simulink model "EPT"  (R2019b)
settings: Solver=FixedStepDiscrete  StartTime=0.0  StopTime=5  FixedStep=0.005  RelTol=1e-3  EnableMultiTasking=on
PreLoadFcn:
  | try, model_open; catch, disp('Error occurred while executing model pre-load callback: model_open.m'); disp('Please assure that the MATLAB working directory is set to the model directory before opening.'); end
InitFcn:
  | try, model_open; catch, end
undefined symbols (not defined in the file or in its folder): Bridge, GCM, H, ln, raptor_get_param_eval, raptor_get_safe_string, raptor_xcp_function
libraries: Raptor_lib x2810, simulink x374, hdlsllib x19
(part 26 of 45)

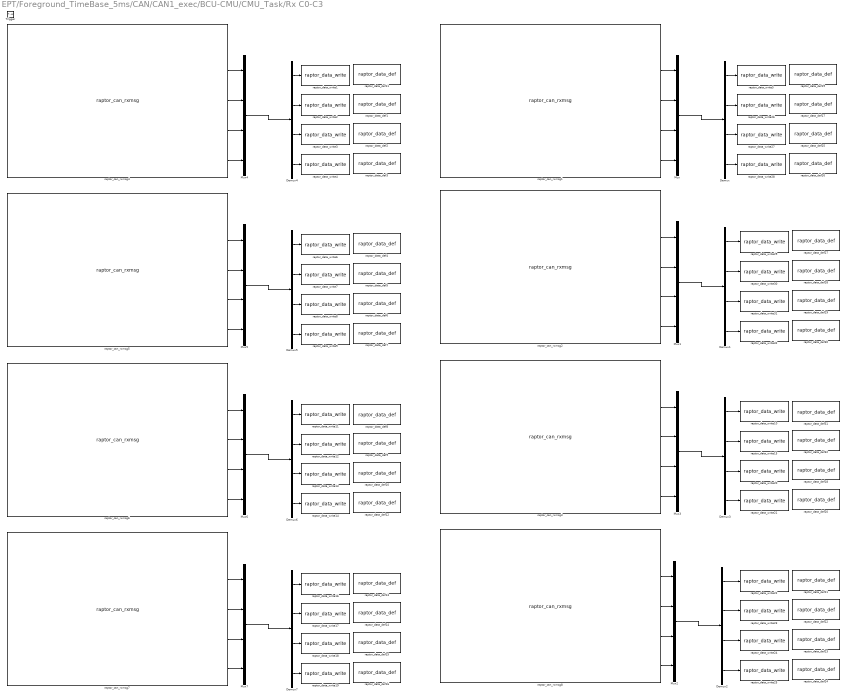
== system EPT/Foreground_TimeBase_5ms/CAN/CAN1_exec/BCU-CMU/CMU_Task/Rx C0-C3 ==
  Trigger : TriggerPort  VariantControl=Variant  PortDimensions=1
  Demux{,1..7} (8 alike) : Demux
  Mux{,1..7} (8 alike) : Mux
  raptor_can_rxmsg1 : Raptor_lib/CAN/raptor_can_rxmsg  canDefinition=struct('dbcFile', 'CMU2.dbc','message', 'Cell_Volt1','comment', '','signals', {{'Vcell1','Vcell2','Vcell3','Vcell4'}},'enabled', [ 1 1 1 1;],'canBus', '''CAN1''','messageID', [ 33603746;],'idMask', [ 536870911;],'payloadMask', [],'payloadValue', [],'period', [ 0;],'mailbox', '''''','queueSize', [ 1;],'label', [ 0;],'ver', [ 2;],'showID', [ 0;],'showRaw', [ 0;],'fill', [ 0;],'editID', [ 0;],'signalOrder', [ 2;])  canBus='CAN1'  mailbox=''  payloadMask=[]  payloadValue=[]  idMask=hex2dec('1FFFFFFF')  queueSize=1  showID=0  label=0  fill=0  id=33603746  showRaw=0  showAge=1  signalOrder=2  signalInfo={{struct('Name', 'Vcell1','Startbit', [ 0;],'SignalSize', [ 16;],'ByteOrder', 'BigEndian','ValueType', 'UNSIGNED','Class', 'uint16','Signed', [ 0;],'Factor', [ 0.001;],'Offset', [ 0;],'Min', [ 0;],'Max', [ 0;],'Units', '','Comment', '','StartBit', [ 8;]),struct('Name', 'Vcell2','Startbit', [ 0;],'SignalSize', [ 16;],'ByteOrder', 'BigEndian','ValueType', 'UNSIGNED','Class', 'uint16','Signed', [ 0;],'Factor', [ 0.001;],'Offset', [ 0;],'Min', [ 0;],'Max', [ 0;],'Units', '','Comment', '','StartBit', [ 24;]),struct('Name', 'Vcell3','Startbit', [ 0;],'SignalSize', [ 16;],'ByteOrder', 'BigEndian','ValueType', 'UNSIGNED','Class', 'uint16','Signed', [ 0;],'Factor', [ 0.001;],'Offset', [ 0;],'Min', [ 0;],'Max', [ 0;],'Units', '','Comment', '','StartBit', [ 40;]),struct('Name', 'Vcell4','Startbit', [ 0;],'SignalSize', [ 16;],'ByteOrder', 'BigEndian','ValueType', 'UNSIGNED','Class', 'uint16','Signed', [ 0;],'Factor', [ 0.001;],'Offset', [ 0;],'Min', [ 0;],'Max', [ 0;],'Units', '','Comment', '','StartBit', [ 56;])}}
      settings: SourceProductName=Raptor
  raptor_can_rxmsg2 : Raptor_lib/CAN/raptor_can_rxmsg  canDefinition=struct('dbcFile', 'CMU2.dbc','message', 'Cell_Volt2','comment', '','signals', {{'Vcell5','Vcell6','Vcell7','Vcell8'}},'enabled', [ 1 1 1 1;],'canBus', '''CAN1''','messageID', [ 33604002;],'idMask', [ 536870911;],'payloadMask', [],'payloadValue', [],'period', [ 0;],'mailbox', '''''','queueSize', [ 1;],'label', [ 0;],'ver', [ 2;],'showID', [ 0;],'showRaw', [ 0;],'fill', [ 0;],'editID', [ 0;],'signalOrder', [ 2;])  canBus='CAN1'  mailbox=''  payloadMask=[]  payloadValue=[]  idMask=hex2dec('1FFFFFFF')  queueSize=1  showID=0  label=0  fill=0  id=33604002  showRaw=0  showAge=1  signalOrder=2  signalInfo={{struct('Name', 'Vcell5','Startbit', [ 0;],'SignalSize', [ 16;],'ByteOrder', 'BigEndian','ValueType', 'UNSIGNED','Class', 'uint16','Signed', [ 0;],'Factor', [ 0.001;],'Offset', [ 0;],'Min', [ 0;],'Max', [ 0;],'Units', '','Comment', '','StartBit', [ 8;]),struct('Name', 'Vcell6','Startbit', [ 0;],'SignalSize', [ 16;],'ByteOrder', 'BigEndian','ValueType', 'UNSIGNED','Class', 'uint16','Signed', [ 0;],'Factor', [ 0.001;],'Offset', [ 0;],'Min', [ 0;],'Max', [ 0;],'Units', '','Comment', '','StartBit', [ 24;]),struct('Name', 'Vcell7','Startbit', [ 0;],'SignalSize', [ 16;],'ByteOrder', 'BigEndian','ValueType', 'UNSIGNED','Class', 'uint16','Signed', [ 0;],'Factor', [ 0.001;],'Offset', [ 0;],'Min', [ 0;],'Max', [ 0;],'Units', '','Comment', '','StartBit', [ 40;]),struct('Name', 'Vcell8','Startbit', [ 0;],'SignalSize', [ 16;],'ByteOrder', 'BigEndian','ValueType', 'UNSIGNED','Class', 'uint16','Signed', [ 0;],'Factor', [ 0.001;],'Offset', [ 0;],'Min', [ 0;],'Max', [ 0;],'Units', '','Comment', '','StartBit', [ 56;])}}
      settings: SourceProductName=Raptor
  raptor_can_rxmsg3 : Raptor_lib/CAN/raptor_can_rxmsg  canDefinition=struct('dbcFile', 'CMU2.dbc','message', 'Cell_Volt3','comment', '','signals', {{'Vcell9','Vcell10','Vcell11','Vcell12'}},'enabled', [ 1 1 1 1;],'canBus', '''CAN1''','messageID', [ 33604258;],'idMask', [ 536870911;],'payloadMask', [],'payloadValue', [],'period', [ 0;],'mailbox', '''''','queueSize', [ 1;],'label', [ 0;],'ver', [ 2;],'showID', [ 0;],'showRaw', [ 0;],'fill', [ 0;],'editID', [ 0;],'signalOrder', [ 2;])  canBus='CAN1'  mailbox=''  payloadMask=[]  payloadValue=[]  idMask=hex2dec('1FFFFFFF')  queueSize=1  showID=0  label=0  fill=0  id=33604258  showRaw=0  showAge=1  signalOrder=2  signalInfo={{struct('Name', 'Vcell9','Startbit', [ 0;],'SignalSize', [ 16;],'ByteOrder', 'BigEndian','ValueType', 'UNSIGNED','Class', 'uint16','Signed', [ 0;],'Factor', [ 0.001;],'Offset', [ 0;],'Min', [ 0;],'Max', [ 0;],'Units', '','Comment', '','StartBit', [ 8;]),struct('Name', 'Vcell10','Startbit', [ 0;],'SignalSize', [ 16;],'ByteOrder', 'BigEndian','ValueType', 'UNSIGNED','Class', 'uint16','Signed', [ 0;],'Factor', [ 0.001;],'Offset', [ 0;],'Min', [ 0;],'Max', [ 0;],'Units', '','Comment', '','StartBit', [ 24;]),struct('Name', 'Vcell11','Startbit', [ 0;],'SignalSize', [ 16;],'ByteOrder', 'BigEndian','ValueType', 'UNSIGNED','Class', 'uint16','Signed', [ 0;],'Factor', [ 0.001;],'Offset', [ 0;],'Min', [ 0;],'Max', [ 0;],'Units', '','Comment', '','StartBit', [ 40;]),struct('Name', 'Vcell12','Startbit', [ 0;],'SignalSize', [ 16;],'ByteOrder', 'BigEndian','ValueType', 'UNSIGNED','Class', 'uint16','Signed', [ 0;],'Factor', [ 0.001;],'Offset', [ 0;],'Min', [ 0;],'Max', [ 0;],'Units', '','Comment', '','StartBit', [ 56;])}}
      settings: SourceProductName=Raptor
  raptor_can_rxmsg4 : Raptor_lib/CAN/raptor_can_rxmsg  canDefinition=struct('dbcFile', 'CMU1.dbc','message', 'Cell_Volt1','comment', '','signals', {{'Vcell1','Vcell2','Vcell3','Vcell4'}},'enabled', [ 1 1 1 1;],'canBus', '''CAN1''','messageID', [ 33603745;],'idMask', [ 536870911;],'payloadMask', [],'payloadValue', [],'period', [ 0;],'mailbox', '''''','queueSize', [ 1;],'label', [ 0;],'ver', [ 2;],'showID', [ 0;],'showRaw', [ 0;],'fill', [ 0;],'editID', [ 0;],'signalOrder', [ 2;])  canBus='CAN1'  mailbox=''  payloadMask=[]  payloadValue=[]  idMask=hex2dec('1FFFFFFF')  queueSize=1  showID=0  label=0  fill=0  id=33603745  showRaw=0  showAge=1  signalOrder=2  signalInfo={{struct('Name', 'Vcell1','Startbit', [ 0;],'SignalSize', [ 16;],'ByteOrder', 'BigEndian','ValueType', 'UNSIGNED','Class', 'uint16','Signed', [ 0;],'Factor', [ 0.001;],'Offset', [ 0;],'Min', [ 0;],'Max', [ 0;],'Units', '','Comment', '','StartBit', [ 8;]),struct('Name', 'Vcell2','Startbit', [ 0;],'SignalSize', [ 16;],'ByteOrder', 'BigEndian','ValueType', 'UNSIGNED','Class', 'uint16','Signed', [ 0;],'Factor', [ 0.001;],'Offset', [ 0;],'Min', [ 0;],'Max', [ 0;],'Units', '','Comment', '','StartBit', [ 24;]),struct('Name', 'Vcell3','Startbit', [ 0;],'SignalSize', [ 16;],'ByteOrder', 'BigEndian','ValueType', 'UNSIGNED','Class', 'uint16','Signed', [ 0;],'Factor', [ 0.001;],'Offset', [ 0;],'Min', [ 0;],'Max', [ 0;],'Units', '','Comment', '','StartBit', [ 40;]),struct('Name', 'Vcell4','Startbit', [ 0;],'SignalSize', [ 16;],'ByteOrder', 'BigEndian','ValueType', 'UNSIGNED','Class', 'uint16','Signed', [ 0;],'Factor', [ 0.001;],'Offset', [ 0;],'Min', [ 0;],'Max', [ 0;],'Units', '','Comment', '','StartBit', [ 56;])}}
      settings: SourceProductName=Raptor
  raptor_can_rxmsg5 : Raptor_lib/CAN/raptor_can_rxmsg  canDefinition=struct('dbcFile', 'CMU1.dbc','message', 'Cell_Volt2','comment', '','signals', {{'Vcell5','Vcell6','Vcell7','Vcell8'}},'enabled', [ 1 1 1 1;],'canBus', '''CAN1''','messageID', [ 33604001;],'idMask', [ 536870911;],'payloadMask', [],'payloadValue', [],'period', [ 0;],'mailbox', '''''','queueSize', [ 1;],'label', [ 0;],'ver', [ 2;],'showID', [ 0;],'showRaw', [ 0;],'fill', [ 0;],'editID', [ 0;],'signalOrder', [ 2;])  canBus='CAN1'  mailbox=''  payloadMask=[]  payloadValue=[]  idMask=hex2dec('1FFFFFFF')  queueSize=1  showID=0  label=0  fill=0  id=33604001  showRaw=0  showAge=1  signalOrder=2  signalInfo={{struct('Name', 'Vcell5','Startbit', [ 0;],'SignalSize', [ 16;],'ByteOrder', 'BigEndian','ValueType', 'UNSIGNED','Class', 'uint16','Signed', [ 0;],'Factor', [ 0.001;],'Offset', [ 0;],'Min', [ 0;],'Max', [ 0;],'Units', '','Comment', '','StartBit', [ 8;]),struct('Name', 'Vcell6','Startbit', [ 0;],'SignalSize', [ 16;],'ByteOrder', 'BigEndian','ValueType', 'UNSIGNED','Class', 'uint16','Signed', [ 0;],'Factor', [ 0.001;],'Offset', [ 0;],'Min', [ 0;],'Max', [ 0;],'Units', '','Comment', '','StartBit', [ 24;]),struct('Name', 'Vcell7','Startbit', [ 0;],'SignalSize', [ 16;],'ByteOrder', 'BigEndian','ValueType', 'UNSIGNED','Class', 'uint16','Signed', [ 0;],'Factor', [ 0.001;],'Offset', [ 0;],'Min', [ 0;],'Max', [ 0;],'Units', '','Comment', '','StartBit', [ 40;]),struct('Name', 'Vcell8','Startbit', [ 0;],'SignalSize', [ 16;],'ByteOrder', 'BigEndian','ValueType', 'UNSIGNED','Class', 'uint16','Signed', [ 0;],'Factor', [ 0.001;],'Offset', [ 0;],'Min', [ 0;],'Max', [ 0;],'Units', '','Comment', '','StartBit', [ 56;])}}
      settings: SourceProductName=Raptor
  raptor_can_rxmsg6 : Raptor_lib/CAN/raptor_can_rxmsg  canDefinition=struct('dbcFile', 'CMU1.dbc','message', 'Cell_Volt3','comment', '','signals', {{'Vcell9','Vcell10','Vcell11','Vcell12'}},'enabled', [ 1 1 1 1;],'canBus', '''CAN1''','messageID', [ 33604257;],'idMask', [ 536870911;],'payloadMask', [],'payloadValue', [],'period', [ 0;],'mailbox', '''''','queueSize', [ 1;],'label', [ 0;],'ver', [ 2;],'showID', [ 0;],'showRaw', [ 0;],'fill', [ 0;],'editID', [ 0;],'signalOrder', [ 3;])  canBus='CAN1'  mailbox=''  payloadMask=[]  payloadValue=[]  idMask=hex2dec('1FFFFFFF')  queueSize=1  showID=0  label=0  fill=0  id=33604257  showRaw=0  showAge=1  signalOrder=3  signalInfo={{struct('Name', 'Vcell9','Startbit', [ 0;],'SignalSize', [ 16;],'ByteOrder', 'BigEndian','ValueType', 'UNSIGNED','Class', 'uint16','Signed', [ 0;],'Factor', [ 0.001;],'Offset', [ 0;],'Min', [ 0;],'Max', [ 0;],'Units', '','Comment', '','StartBit', [ 8;]),struct('Name', 'Vcell10','Startbit', [ 0;],'SignalSize', [ 16;],'ByteOrder', 'BigEndian','ValueType', 'UNSIGNED','Class', 'uint16','Signed', [ 0;],'Factor', [ 0.001;],'Offset', [ 0;],'Min', [ 0;],'Max', [ 0;],'Units', '','Comment', '','StartBit', [ 24;]),struct('Name', 'Vcell11','Startbit', [ 0;],'SignalSize', [ 16;],'ByteOrder', 'BigEndian','ValueType', 'UNSIGNED','Class', 'uint16','Signed', [ 0;],'Factor', [ 0.001;],'Offset', [ 0;],'Min', [ 0;],'Max', [ 0;],'Units', '','Comment', '','StartBit', [ 40;]),struct('Name', 'Vcell12','Startbit', [ 0;],'SignalSize', [ 16;],'ByteOrder', 'BigEndian','ValueType', 'UNSIGNED','Class', 'uint16','Signed', [ 0;],'Factor', [ 0.001;],'Offset', [ 0;],'Min', [ 0;],'Max', [ 0;],'Units', '','Comment', '','StartBit', [ 56;])}}
      settings: SourceProductName=Raptor
  raptor_can_rxmsg7 : Raptor_lib/CAN/raptor_can_rxmsg  canDefinition=struct('dbcFile', 'CMU1.dbc','message', 'Cell_Volt4','comment', '','signals', {{'Vcell13','Vcell14','Vcell15','Vcell16'}},'enabled', [ 1 1 1 1;],'canBus', '''CAN1''','messageID', [ 33604513;],'idMask', [ 536870911;],'payloadMask', [],'payloadValue', [],'period', [ 0;],'mailbox', '''''','queueSize', [ 1;],'label', [ 0;],'ver', [ 2;],'showID', [ 0;],'showRaw', [ 0;],'fill', [ 0;],'editID', [ 0;],'signalOrder', [ 2;])  canBus='CAN1'  mailbox=''  payloadMask=[]  payloadValue=[]  idMask=hex2dec('1FFFFFFF')  queueSize=1  showID=0  label=0  fill=0  id=33604513  showRaw=0  showAge=1  signalOrder=2  signalInfo={{struct('Name', 'Vcell13','Startbit', [ 0;],'SignalSize', [ 16;],'ByteOrder', 'BigEndian','ValueType', 'UNSIGNED','Class', 'uint16','Signed', [ 0;],'Factor', [ 0.001;],'Offset', [ 0;],'Min', [ 0;],'Max', [ 0;],'Units', '','Comment', '','StartBit', [ 8;]),struct('Name', 'Vcell14','Startbit', [ 0;],'SignalSize', [ 16;],'ByteOrder', 'BigEndian','ValueType', 'UNSIGNED','Class', 'uint16','Signed', [ 0;],'Factor', [ 0.001;],'Offset', [ 0;],'Min', [ 0;],'Max', [ 0;],'Units', '','Comment', '','StartBit', [ 24;]),struct('Name', 'Vcell15','Startbit', [ 0;],'SignalSize', [ 16;],'ByteOrder', 'BigEndian','ValueType', 'UNSIGNED','Class', 'uint16','Signed', [ 0;],'Factor', [ 0.001;],'Offset', [ 0;],'Min', [ 0;],'Max', [ 0;],'Units', '','Comment', '','StartBit', [ 40;]),struct('Name', 'Vcell16','Startbit', [ 0;],'SignalSize', [ 16;],'ByteOrder', 'BigEndian','ValueType', 'UNSIGNED','Class', 'uint16','Signed', [ 0;],'Factor', [ 0.001;],'Offset', [ 0;],'Min', [ 0;],'Max', [ 0;],'Units', '','Comment', '','StartBit', [ 56;])}}
      settings: SourceProductName=Raptor
  raptor_can_rxmsg8 : Raptor_lib/CAN/raptor_can_rxmsg  canDefinition=struct('dbcFile', 'CMU2.dbc','message', 'Cell_Volt4','comment', '','signals', {{'Vcell13','Vcell14','Vcell15','Vcell16'}},'enabled', [ 1 1 1 1;],'canBus', '''CAN1''','messageID', [ 33604514;],'idMask', [ 536870911;],'payloadMask', [],'payloadValue', [],'period', [ 0;],'mailbox', '''''','queueSize', [ 1;],'label', [ 0;],'ver', [ 2;],'showID', [ 0;],'showRaw', [ 0;],'fill', [ 0;],'editID', [ 0;],'signalOrder', [ 2;])  canBus='CAN1'  mailbox=''  payloadMask=[]  payloadValue=[]  idMask=hex2dec('1FFFFFFF')  queueSize=1  showID=0  label=0  fill=0  id=33604514  showRaw=0  showAge=1  signalOrder=2  signalInfo={{struct('Name', 'Vcell13','Startbit', [ 0;],'SignalSize', [ 16;],'ByteOrder', 'BigEndian','ValueType', 'UNSIGNED','Class', 'uint16','Signed', [ 0;],'Factor', [ 0.001;],'Offset', [ 0;],'Min', [ 0;],'Max', [ 0;],'Units', '','Comment', '','StartBit', [ 8;]),struct('Name', 'Vcell14','Startbit', [ 0;],'SignalSize', [ 16;],'ByteOrder', 'BigEndian','ValueType', 'UNSIGNED','Class', 'uint16','Signed', [ 0;],'Factor', [ 0.001;],'Offset', [ 0;],'Min', [ 0;],'Max', [ 0;],'Units', '','Comment', '','StartBit', [ 24;]),struct('Name', 'Vcell15','Startbit', [ 0;],'SignalSize', [ 16;],'ByteOrder', 'BigEndian','ValueType', 'UNSIGNED','Class', 'uint16','Signed', [ 0;],'Factor', [ 0.001;],'Offset', [ 0;],'Min', [ 0;],'Max', [ 0;],'Units', '','Comment', '','StartBit', [ 40;]),struct('Name', 'Vcell16','Startbit', [ 0;],'SignalSize', [ 16;],'ByteOrder', 'BigEndian','ValueType', 'UNSIGNED','Class', 'uint16','Signed', [ 0;],'Factor', [ 0.001;],'Offset', [ 0;],'Min', [ 0;],'Max', [ 0;],'Units', '','Comment', '','StartBit', [ 56;])}}
      settings: SourceProductName=Raptor
  raptor_data_def1 : Raptor_lib/Data Storage/raptor_data_def  dataName='CMU1_CELL02_VOLT'  initValue=0  dataType=double  storage=Volatile (RAM)  calVisible=on  calType=Adjustment  calDispType=Number  calEnum={'False', 'True'}  calGain=1.0  calOffset=0  calMin=-inf  calMax=inf  calFormat='2.3'  calUnit=''  calHelp=''  calAccess=1  calFunction=raptor_xcp_function(gcb)  calDispHeaders=off  calColHeaders={'Col1' 'Col2' 'Col3'}  calRowHeaders={'Row1' 'Row2' 'Row3'}
      settings: SourceProductName=Raptor
  raptor_data_def10 : Raptor_lib/Data Storage/raptor_data_def  dataName='CMU1_CELL11_VOLT'  initValue=0  dataType=double  storage=Volatile (RAM)  calVisible=on  calType=Adjustment  calDispType=Number  calEnum={'False', 'True'}  calGain=1.0  calOffset=0  calMin=-inf  calMax=inf  calFormat='2.3'  calUnit=''  calHelp=''  calAccess=1  calFunction=raptor_xcp_function(gcb)  calDispHeaders=off  calColHeaders={'Col1' 'Col2' 'Col3'}  calRowHeaders={'Row1' 'Row2' 'Row3'}
      settings: SourceProductName=Raptor
  raptor_data_def11 : Raptor_lib/Data Storage/raptor_data_def  dataName='CMU1_CELL01_VOLT'  initValue=0  dataType=double  storage=Volatile (RAM)  calVisible=on  calType=Adjustment  calDispType=Number  calEnum={'False', 'True'}  calGain=1.0  calOffset=0  calMin=-inf  calMax=inf  calFormat='2.3'  calUnit=''  calHelp=''  calAccess=1  calFunction=raptor_xcp_function(gcb)  calDispHeaders=off  calColHeaders={'Col1' 'Col2' 'Col3'}  calRowHeaders={'Row1' 'Row2' 'Row3'}
      settings: SourceProductName=Raptor
  raptor_data_def12 : Raptor_lib/Data Storage/raptor_data_def  dataName='CMU1_CELL12_VOLT'  initValue=0  dataType=double  storage=Volatile (RAM)  calVisible=on  calType=Adjustment  calDispType=Number  calEnum={'False', 'True'}  calGain=1.0  calOffset=0  calMin=-inf  calMax=inf  calFormat='2.3'  calUnit=''  calHelp=''  calAccess=1  calFunction=raptor_xcp_function(gcb)  calDispHeaders=off  calColHeaders={'Col1' 'Col2' 'Col3'}  calRowHeaders={'Row1' 'Row2' 'Row3'}
      settings: SourceProductName=Raptor
  raptor_data_def13 : Raptor_lib/Data Storage/raptor_data_def  dataName='CMU1_CELL13_VOLT'  initValue=0  dataType=double  storage=Volatile (RAM)  calVisible=on  calType=Adjustment  calDispType=Number  calEnum={'False', 'True'}  calGain=1.0  calOffset=0  calMin=-inf  calMax=inf  calFormat='2.3'  calUnit=''  calHelp=''  calAccess=1  calFunction=raptor_xcp_function(gcb)  calDispHeaders=off  calColHeaders={'Col1' 'Col2' 'Col3'}  calRowHeaders={'Row1' 'Row2' 'Row3'}
      settings: SourceProductName=Raptor
  raptor_data_def14 : Raptor_lib/Data Storage/raptor_data_def  dataName='CMU1_CELL14_VOLT'  initValue=0  dataType=double  storage=Volatile (RAM)  calVisible=on  calType=Adjustment  calDispType=Number  calEnum={'False', 'True'}  calGain=1.0  calOffset=0  calMin=-inf  calMax=inf  calFormat='2.3'  calUnit=''  calHelp=''  calAccess=1  calFunction=raptor_xcp_function(gcb)  calDispHeaders=off  calColHeaders={'Col1' 'Col2' 'Col3'}  calRowHeaders={'Row1' 'Row2' 'Row3'}
      settings: SourceProductName=Raptor
  raptor_data_def15 : Raptor_lib/Data Storage/raptor_data_def  dataName='CMU1_CELL15_VOLT'  initValue=0  dataType=double  storage=Volatile (RAM)  calVisible=on  calType=Adjustment  calDispType=Number  calEnum={'False', 'True'}  calGain=1.0  calOffset=0  calMin=-inf  calMax=inf  calFormat='2.3'  calUnit=''  calHelp=''  calAccess=1  calFunction=raptor_xcp_function(gcb)  calDispHeaders=off  calColHeaders={'Col1' 'Col2' 'Col3'}  calRowHeaders={'Row1' 'Row2' 'Row3'}
      settings: SourceProductName=Raptor
  raptor_data_def16 : Raptor_lib/Data Storage/raptor_data_def  dataName='CMU1_CELL16_VOLT'  initValue=0  dataType=double  storage=Volatile (RAM)  calVisible=on  calType=Adjustment  calDispType=Number  calEnum={'False', 'True'}  calGain=1.0  calOffset=0  calMin=-inf  calMax=inf  calFormat='2.3'  calUnit=''  calHelp=''  calAccess=1  calFunction=raptor_xcp_function(gcb)  calDispHeaders=off  calColHeaders={'Col1' 'Col2' 'Col3'}  calRowHeaders={'Row1' 'Row2' 'Row3'}
      settings: SourceProductName=Raptor
  raptor_data_def17 : Raptor_lib/Data Storage/raptor_data_def  dataName='CMU2_CELL02_VOLT'  initValue=0  dataType=double  storage=Volatile (RAM)  calVisible=on  calType=Adjustment  calDispType=Number  calEnum={'False', 'True'}  calGain=1.0  calOffset=0  calMin=-inf  calMax=inf  calFormat='2.3'  calUnit=''  calHelp=''  calAccess=1  calFunction=raptor_xcp_function(gcb)  calDispHeaders=off  calColHeaders={'Col1' 'Col2' 'Col3'}  calRowHeaders={'Row1' 'Row2' 'Row3'}
      settings: SourceProductName=Raptor
  raptor_data_def18 : Raptor_lib/Data Storage/raptor_data_def  dataName='CMU2_CELL11_VOLT'  initValue=0  dataType=double  storage=Volatile (RAM)  calVisible=on  calType=Adjustment  calDispType=Number  calEnum={'False', 'True'}  calGain=1.0  calOffset=0  calMin=-inf  calMax=inf  calFormat='2.3'  calUnit=''  calHelp=''  calAccess=1  calFunction=raptor_xcp_function(gcb)  calDispHeaders=off  calColHeaders={'Col1' 'Col2' 'Col3'}  calRowHeaders={'Row1' 'Row2' 'Row3'}
      settings: SourceProductName=Raptor
  raptor_data_def19 : Raptor_lib/Data Storage/raptor_data_def  dataName='CMU2_CELL01_VOLT'  initValue=0  dataType=double  storage=Volatile (RAM)  calVisible=on  calType=Adjustment  calDispType=Number  calEnum={'False', 'True'}  calGain=1.0  calOffset=0  calMin=-inf  calMax=inf  calFormat='2.3'  calUnit=''  calHelp=''  calAccess=1  calFunction=raptor_xcp_function(gcb)  calDispHeaders=off  calColHeaders={'Col1' 'Col2' 'Col3'}  calRowHeaders={'Row1' 'Row2' 'Row3'}
      settings: SourceProductName=Raptor
  raptor_data_def2 : Raptor_lib/Data Storage/raptor_data_def  dataName='CMU1_CELL03_VOLT'  initValue=0  dataType=double  storage=Volatile (RAM)  calVisible=on  calType=Adjustment  calDispType=Number  calEnum={'False', 'True'}  calGain=1.0  calOffset=0  calMin=-inf  calMax=inf  calFormat='2.3'  calUnit=''  calHelp=''  calAccess=1  calFunction=raptor_xcp_function(gcb)  calDispHeaders=off  calColHeaders={'Col1' 'Col2' 'Col3'}  calRowHeaders={'Row1' 'Row2' 'Row3'}
      settings: SourceProductName=Raptor
  raptor_data_def20 : Raptor_lib/Data Storage/raptor_data_def  dataName='CMU2_CELL12_VOLT'  initValue=0  dataType=double  storage=Volatile (RAM)  calVisible=on  calType=Adjustment  calDispType=Number  calEnum={'False', 'True'}  calGain=1.0  calOffset=0  calMin=-inf  calMax=inf  calFormat='2.3'  calUnit=''  calHelp=''  calAccess=1  calFunction=raptor_xcp_function(gcb)  calDispHeaders=off  calColHeaders={'Col1' 'Col2' 'Col3'}  calRowHeaders={'Row1' 'Row2' 'Row3'}
      settings: SourceProductName=Raptor
  raptor_data_def21 : Raptor_lib/Data Storage/raptor_data_def  dataName='CMU2_CELL13_VOLT'  initValue=0  dataType=double  storage=Volatile (RAM)  calVisible=on  calType=Adjustment  calDispType=Number  calEnum={'False', 'True'}  calGain=1.0  calOffset=0  calMin=-inf  calMax=inf  calFormat='2.3'  calUnit=''  calHelp=''  calAccess=1  calFunction=raptor_xcp_function(gcb)  calDispHeaders=off  calColHeaders={'Col1' 'Col2' 'Col3'}  calRowHeaders={'Row1' 'Row2' 'Row3'}
      settings: SourceProductName=Raptor
  raptor_data_def22 : Raptor_lib/Data Storage/raptor_data_def  dataName='CMU2_CELL14_VOLT'  initValue=0  dataType=double  storage=Volatile (RAM)  calVisible=on  calType=Adjustment  calDispType=Number  calEnum={'False', 'True'}  calGain=1.0  calOffset=0  calMin=-inf  calMax=inf  calFormat='2.3'  calUnit=''  calHelp=''  calAccess=1  calFunction=raptor_xcp_function(gcb)  calDispHeaders=off  calColHeaders={'Col1' 'Col2' 'Col3'}  calRowHeaders={'Row1' 'Row2' 'Row3'}
      settings: SourceProductName=Raptor
  raptor_data_def23 : Raptor_lib/Data Storage/raptor_data_def  dataName='CMU2_CELL15_VOLT'  initValue=0  dataType=double  storage=Volatile (RAM)  calVisible=on  calType=Adjustment  calDispType=Number  calEnum={'False', 'True'}  calGain=1.0  calOffset=0  calMin=-inf  calMax=inf  calFormat='2.3'  calUnit=''  calHelp=''  calAccess=1  calFunction=raptor_xcp_function(gcb)  calDispHeaders=off  calColHeaders={'Col1' 'Col2' 'Col3'}  calRowHeaders={'Row1' 'Row2' 'Row3'}
      settings: SourceProductName=Raptor
  raptor_data_def24 : Raptor_lib/Data Storage/raptor_data_def  dataName='CMU2_CELL16_VOLT'  initValue=0  dataType=double  storage=Volatile (RAM)  calVisible=on  calType=Adjustment  calDispType=Number  calEnum={'False', 'True'}  calGain=1.0  calOffset=0  calMin=-inf  calMax=inf  calFormat='2.3'  calUnit=''  calHelp=''  calAccess=1  calFunction=raptor_xcp_function(gcb)  calDispHeaders=off  calColHeaders={'Col1' 'Col2' 'Col3'}  calRowHeaders={'Row1' 'Row2' 'Row3'}
      settings: SourceProductName=Raptor
  raptor_data_def25 : Raptor_lib/Data Storage/raptor_data_def  dataName='CMU2_CELL03_VOLT'  initValue=0  dataType=double  storage=Volatile (RAM)  calVisible=on  calType=Adjustment  calDispType=Number  calEnum={'False', 'True'}  calGain=1.0  calOffset=0  calMin=-inf  calMax=inf  calFormat='2.3'  calUnit=''  calHelp=''  calAccess=1  calFunction=raptor_xcp_function(gcb)  calDispHeaders=off  calColHeaders={'Col1' 'Col2' 'Col3'}  calRowHeaders={'Row1' 'Row2' 'Row3'}
      settings: SourceProductName=Raptor
  raptor_data_def26 : Raptor_lib/Data Storage/raptor_data_def  dataName='CMU2_CELL04_VOLT'  initValue=0  dataType=double  storage=Volatile (RAM)  calVisible=on  calType=Adjustment  calDispType=Number  calEnum={'False', 'True'}  calGain=1.0  calOffset=0  calMin=-inf  calMax=inf  calFormat='2.3'  calUnit=''  calHelp=''  calAccess=1  calFunction=raptor_xcp_function(gcb)  calDispHeaders=off  calColHeaders={'Col1' 'Col2' 'Col3'}  calRowHeaders={'Row1' 'Row2' 'Row3'}
      settings: SourceProductName=Raptor
  raptor_data_def27 : Raptor_lib/Data Storage/raptor_data_def  dataName='CMU2_CELL05_VOLT'  initValue=0  dataType=double  storage=Volatile (RAM)  calVisible=on  calType=Adjustment  calDispType=Number  calEnum={'False', 'True'}  calGain=1.0  calOffset=0  calMin=-inf  calMax=inf  calFormat='2.3'  calUnit=''  calHelp=''  calAccess=1  calFunction=raptor_xcp_function(gcb)  calDispHeaders=off  calColHeaders={'Col1' 'Col2' 'Col3'}  calRowHeaders={'Row1' 'Row2' 'Row3'}
      settings: SourceProductName=Raptor
  raptor_data_def28 : Raptor_lib/Data Storage/raptor_data_def  dataName='CMU2_CELL06_VOLT'  initValue=0  dataType=double  storage=Volatile (RAM)  calVisible=on  calType=Adjustment  calDispType=Number  calEnum={'False', 'True'}  calGain=1.0  calOffset=0  calMin=-inf  calMax=inf  calFormat='2.3'  calUnit=''  calHelp=''  calAccess=1  calFunction=raptor_xcp_function(gcb)  calDispHeaders=off  calColHeaders={'Col1' 'Col2' 'Col3'}  calRowHeaders={'Row1' 'Row2' 'Row3'}
      settings: SourceProductName=Raptor
  raptor_data_def29 : Raptor_lib/Data Storage/raptor_data_def  dataName='CMU2_CELL07_VOLT'  initValue=0  dataType=double  storage=Volatile (RAM)  calVisible=on  calType=Adjustment  calDispType=Number  calEnum={'False', 'True'}  calGain=1.0  calOffset=0  calMin=-inf  calMax=inf  calFormat='2.3'  calUnit=''  calHelp=''  calAccess=1  calFunction=raptor_xcp_function(gcb)  calDispHeaders=off  calColHeaders={'Col1' 'Col2' 'Col3'}  calRowHeaders={'Row1' 'Row2' 'Row3'}
      settings: SourceProductName=Raptor
  raptor_data_def3 : Raptor_lib/Data Storage/raptor_data_def  dataName='CMU1_CELL04_VOLT'  initValue=0  dataType=double  storage=Volatile (RAM)  calVisible=on  calType=Adjustment  calDispType=Number  calEnum={'False', 'True'}  calGain=1.0  calOffset=0  calMin=-inf  calMax=inf  calFormat='2.3'  calUnit=''  calHelp=''  calAccess=1  calFunction=raptor_xcp_function(gcb)  calDispHeaders=off  calColHeaders={'Col1' 'Col2' 'Col3'}  calRowHeaders={'Row1' 'Row2' 'Row3'}
      settings: SourceProductName=Raptor
  raptor_data_def30 : Raptor_lib/Data Storage/raptor_data_def  dataName='CMU2_CELL08_VOLT'  initValue=0  dataType=double  storage=Volatile (RAM)  calVisible=on  calType=Adjustment  calDispType=Number  calEnum={'False', 'True'}  calGain=1.0  calOffset=0  calMin=-inf  calMax=inf  calFormat='2.3'  calUnit=''  calHelp=''  calAccess=1  calFunction=raptor_xcp_function(gcb)  calDispHeaders=off  calColHeaders={'Col1' 'Col2' 'Col3'}  calRowHeaders={'Row1' 'Row2' 'Row3'}
      settings: SourceProductName=Raptor
  raptor_data_def31 : Raptor_lib/Data Storage/raptor_data_def  dataName='CMU2_CELL09_VOLT'  initValue=0  dataType=double  storage=Volatile (RAM)  calVisible=on  calType=Adjustment  calDispType=Number  calEnum={'False', 'True'}  calGain=1.0  calOffset=0  calMin=-inf  calMax=inf  calFormat='2.3'  calUnit=''  calHelp=''  calAccess=1  calFunction=raptor_xcp_function(gcb)  calDispHeaders=off  calColHeaders={'Col1' 'Col2' 'Col3'}  calRowHeaders={'Row1' 'Row2' 'Row3'}
      settings: SourceProductName=Raptor
  raptor_data_def32 : Raptor_lib/Data Storage/raptor_data_def  dataName='CMU2_CELL10_VOLT'  initValue=0  dataType=double  storage=Volatile (RAM)  calVisible=on  calType=Adjustment  calDispType=Number  calEnum={'False', 'True'}  calGain=1.0  calOffset=0  calMin=-inf  calMax=inf  calFormat='2.3'  calUnit=''  calHelp=''  calAccess=1  calFunction=raptor_xcp_function(gcb)  calDispHeaders=off  calColHeaders={'Col1' 'Col2' 'Col3'}  calRowHeaders={'Row1' 'Row2' 'Row3'}
      settings: SourceProductName=Raptor
  raptor_data_def4 : Raptor_lib/Data Storage/raptor_data_def  dataName='CMU1_CELL05_VOLT'  initValue=0  dataType=double  storage=Volatile (RAM)  calVisible=on  calType=Adjustment  calDispType=Number  calEnum={'False', 'True'}  calGain=1.0  calOffset=0  calMin=-inf  calMax=inf  calFormat='2.3'  calUnit=''  calHelp=''  calAccess=1  calFunction=raptor_xcp_function(gcb)  calDispHeaders=off  calColHeaders={'Col1' 'Col2' 'Col3'}  calRowHeaders={'Row1' 'Row2' 'Row3'}
      settings: SourceProductName=Raptor
  raptor_data_def5 : Raptor_lib/Data Storage/raptor_data_def  dataName='CMU1_CELL06_VOLT'  initValue=0  dataType=double  storage=Volatile (RAM)  calVisible=on  calType=Adjustment  calDispType=Number  calEnum={'False', 'True'}  calGain=1.0  calOffset=0  calMin=-inf  calMax=inf  calFormat='2.3'  calUnit=''  calHelp=''  calAccess=1  calFunction=raptor_xcp_function(gcb)  calDispHeaders=off  calColHeaders={'Col1' 'Col2' 'Col3'}  calRowHeaders={'Row1' 'Row2' 'Row3'}
      settings: SourceProductName=Raptor
  raptor_data_def6 : Raptor_lib/Data Storage/raptor_data_def  dataName='CMU1_CELL07_VOLT'  initValue=0  dataType=double  storage=Volatile (RAM)  calVisible=on  calType=Adjustment  calDispType=Number  calEnum={'False', 'True'}  calGain=1.0  calOffset=0  calMin=-inf  calMax=inf  calFormat='2.3'  calUnit=''  calHelp=''  calAccess=1  calFunction=raptor_xcp_function(gcb)  calDispHeaders=off  calColHeaders={'Col1' 'Col2' 'Col3'}  calRowHeaders={'Row1' 'Row2' 'Row3'}
      settings: SourceProductName=Raptor
  raptor_data_def7 : Raptor_lib/Data Storage/raptor_data_def  dataName='CMU1_CELL08_VOLT'  initValue=0  dataType=double  storage=Volatile (RAM)  calVisible=on  calType=Adjustment  calDispType=Number  calEnum={'False', 'True'}  calGain=1.0  calOffset=0  calMin=-inf  calMax=inf  calFormat='2.3'  calUnit=''  calHelp=''  calAccess=1  calFunction=raptor_xcp_function(gcb)  calDispHeaders=off  calColHeaders={'Col1' 'Col2' 'Col3'}  calRowHeaders={'Row1' 'Row2' 'Row3'}
      settings: SourceProductName=Raptor
  raptor_data_def8 : Raptor_lib/Data Storage/raptor_data_def  dataName='CMU1_CELL09_VOLT'  initValue=0  dataType=double  storage=Volatile (RAM)  calVisible=on  calType=Adjustment  calDispType=Number  calEnum={'False', 'True'}  calGain=1.0  calOffset=0  calMin=-inf  calMax=inf  calFormat='2.3'  calUnit=''  calHelp=''  calAccess=1  calFunction=raptor_xcp_function(gcb)  calDispHeaders=off  calColHeaders={'Col1' 'Col2' 'Col3'}  calRowHeaders={'Row1' 'Row2' 'Row3'}
      settings: SourceProductName=Raptor
  raptor_data_def9 : Raptor_lib/Data Storage/raptor_data_def  dataName='CMU1_CELL10_VOLT'  initValue=0  dataType=double  storage=Volatile (RAM)  calVisible=on  calType=Adjustment  calDispType=Number  calEnum={'False', 'True'}  calGain=1.0  calOffset=0  calMin=-inf  calMax=inf  calFormat='2.3'  calUnit=''  calHelp=''  calAccess=1  calFunction=raptor_xcp_function(gcb)  calDispHeaders=off  calColHeaders={'Col1' 'Col2' 'Col3'}  calRowHeaders={'Row1' 'Row2' 'Row3'}
      settings: SourceProductName=Raptor
  raptor_data_write1 : Raptor_lib/Data Storage/raptor_data_write  dataName='CMU1_CELL01_VOLT'  dataShape=Scalar  idxSource=Input Port  idxRow=1  idxCol=1
      settings: SourceProductName=Raptor
  raptor_data_write10 : Raptor_lib/Data Storage/raptor_data_write  dataName='CMU2_CELL09_VOLT'  dataShape=Scalar  idxSource=Input Port  idxRow=1  idxCol=1
      settings: SourceProductName=Raptor
  raptor_data_write11 : Raptor_lib/Data Storage/raptor_data_write  dataName='CMU1_CELL09_VOLT'  dataShape=Scalar  idxSource=Input Port  idxRow=1  idxCol=1
      settings: SourceProductName=Raptor
  raptor_data_write12 : Raptor_lib/Data Storage/raptor_data_write  dataName='CMU1_CELL10_VOLT'  dataShape=Scalar  idxSource=Input Port  idxRow=1  idxCol=1
      settings: SourceProductName=Raptor
  raptor_data_write13 : Raptor_lib/Data Storage/raptor_data_write  dataName='CMU1_CELL11_VOLT'  dataShape=Scalar  idxSource=Input Port  idxRow=1  idxCol=1
      settings: SourceProductName=Raptor
  raptor_data_write14 : Raptor_lib/Data Storage/raptor_data_write  dataName='CMU1_CELL12_VOLT'  dataShape=Scalar  idxSource=Input Port  idxRow=1  idxCol=1
      settings: SourceProductName=Raptor
  raptor_data_write15 : Raptor_lib/Data Storage/raptor_data_write  dataName='CMU2_CELL10_VOLT'  dataShape=Scalar  idxSource=Input Port  idxRow=1  idxCol=1
      settings: SourceProductName=Raptor
  raptor_data_write16 : Raptor_lib/Data Storage/raptor_data_write  dataName='CMU1_CELL13_VOLT'  dataShape=Scalar  idxSource=Input Port  idxRow=1  idxCol=1
      settings: SourceProductName=Raptor
  raptor_data_write17 : Raptor_lib/Data Storage/raptor_data_write  dataName='CMU1_CELL14_VOLT'  dataShape=Scalar  idxSource=Input Port  idxRow=1  idxCol=1
      settings: SourceProductName=Raptor
  raptor_data_write18 : Raptor_lib/Data Storage/raptor_data_write  dataName='CMU1_CELL15_VOLT'  dataShape=Scalar  idxSource=Input Port  idxRow=1  idxCol=1
      settings: SourceProductName=Raptor
  raptor_data_write19 : Raptor_lib/Data Storage/raptor_data_write  dataName='CMU1_CELL16_VOLT'  dataShape=Scalar  idxSource=Input Port  idxRow=1  idxCol=1
      settings: SourceProductName=Raptor
  raptor_data_write2 : Raptor_lib/Data Storage/raptor_data_write  dataName='CMU1_CELL02_VOLT'  dataShape=Scalar  idxSource=Input Port  idxRow=1  idxCol=1
      settings: SourceProductName=Raptor
  raptor_data_write20 : Raptor_lib/Data Storage/raptor_data_write  dataName='CMU2_CELL11_VOLT'  dataShape=Scalar  idxSource=Input Port  idxRow=1  idxCol=1
      settings: SourceProductName=Raptor
  raptor_data_write21 : Raptor_lib/Data Storage/raptor_data_write  dataName='CMU2_CELL12_VOLT'  dataShape=Scalar  idxSource=Input Port  idxRow=1  idxCol=1
      settings: SourceProductName=Raptor
  raptor_data_write22 : Raptor_lib/Data Storage/raptor_data_write  dataName='CMU2_CELL13_VOLT'  dataShape=Scalar  idxSource=Input Port  idxRow=1  idxCol=1
      settings: SourceProductName=Raptor
  raptor_data_write23 : Raptor_lib/Data Storage/raptor_data_write  dataName='CMU2_CELL14_VOLT'  dataShape=Scalar  idxSource=Input Port  idxRow=1  idxCol=1
      settings: SourceProductName=Raptor
  raptor_data_write24 : Raptor_lib/Data Storage/raptor_data_write  dataName='CMU2_CELL15_VOLT'  dataShape=Scalar  idxSource=Input Port  idxRow=1  idxCol=1
      settings: SourceProductName=Raptor
  raptor_data_write25 : Raptor_lib/Data Storage/raptor_data_write  dataName='CMU2_CELL16_VOLT'  dataShape=Scalar  idxSource=Input Port  idxRow=1  idxCol=1
      settings: SourceProductName=Raptor
  raptor_data_write26 : Raptor_lib/Data Storage/raptor_data_write  dataName='CMU2_CELL02_VOLT'  dataShape=Scalar  idxSource=Input Port  idxRow=1  idxCol=1
      settings: SourceProductName=Raptor
  raptor_data_write27 : Raptor_lib/Data Storage/raptor_data_write  dataName='CMU2_CELL03_VOLT'  dataShape=Scalar  idxSource=Input Port  idxRow=1  idxCol=1
      settings: SourceProductName=Raptor
  raptor_data_write28 : Raptor_lib/Data Storage/raptor_data_write  dataName='CMU2_CELL04_VOLT'  dataShape=Scalar  idxSource=Input Port  idxRow=1  idxCol=1
      settings: SourceProductName=Raptor
  raptor_data_write29 : Raptor_lib/Data Storage/raptor_data_write  dataName='CMU2_CELL05_VOLT'  dataShape=Scalar  idxSource=Input Port  idxRow=1  idxCol=1
      settings: SourceProductName=Raptor
  raptor_data_write3 : Raptor_lib/Data Storage/raptor_data_write  dataName='CMU1_CELL03_VOLT'  dataShape=Scalar  idxSource=Input Port  idxRow=1  idxCol=1
      settings: SourceProductName=Raptor
  raptor_data_write30 : Raptor_lib/Data Storage/raptor_data_write  dataName='CMU2_CELL06_VOLT'  dataShape=Scalar  idxSource=Input Port  idxRow=1  idxCol=1
      settings: SourceProductName=Raptor
  raptor_data_write31 : Raptor_lib/Data Storage/raptor_data_write  dataName='CMU2_CELL07_VOLT'  dataShape=Scalar  idxSource=Input Port  idxRow=1  idxCol=1
      settings: SourceProductName=Raptor
  raptor_data_write32 : Raptor_lib/Data Storage/raptor_data_write  dataName='CMU2_CELL08_VOLT'  dataShape=Scalar  idxSource=Input Port  idxRow=1  idxCol=1
      settings: SourceProductName=Raptor
  raptor_data_write4 : Raptor_lib/Data Storage/raptor_data_write  dataName='CMU1_CELL04_VOLT'  dataShape=Scalar  idxSource=Input Port  idxRow=1  idxCol=1
      settings: SourceProductName=Raptor
  raptor_data_write5 : Raptor_lib/Data Storage/raptor_data_write  dataName='CMU2_CELL01_VOLT'  dataShape=Scalar  idxSource=Input Port  idxRow=1  idxCol=1
      settings: SourceProductName=Raptor
  raptor_data_write6 : Raptor_lib/Data Storage/raptor_data_write  dataName='CMU1_CELL05_VOLT'  dataShape=Scalar  idxSource=Input Port  idxRow=1  idxCol=1
      settings: SourceProductName=Raptor
  raptor_data_write7 : Raptor_lib/Data Storage/raptor_data_write  dataName='CMU1_CELL06_VOLT'  dataShape=Scalar  idxSource=Input Port  idxRow=1  idxCol=1
      settings: SourceProductName=Raptor
  raptor_data_write8 : Raptor_lib/Data Storage/raptor_data_write  dataName='CMU1_CELL07_VOLT'  dataShape=Scalar  idxSource=Input Port  idxRow=1  idxCol=1
      settings: SourceProductName=Raptor
  raptor_data_write9 : Raptor_lib/Data Storage/raptor_data_write  dataName='CMU1_CELL08_VOLT'  dataShape=Scalar  idxSource=Input Port  idxRow=1  idxCol=1
      settings: SourceProductName=Raptor
  wires:
  Mux/1 -> Demux/1
  raptor_can_rxmsg1/5 -> Mux/4
  raptor_can_rxmsg1/4 -> Mux/3
  raptor_can_rxmsg1/3 -> Mux/2
  raptor_can_rxmsg1/2 -> Mux/1
  Demux/1 -> raptor_data_write5/1
  Demux/4 -> raptor_data_write28/1
  Demux/3 -> raptor_data_write27/1
  Demux/2 -> raptor_data_write26/1
  Demux1/2 -> raptor_data_write30/1
  raptor_can_rxmsg2/4 -> Mux1/3
  raptor_can_rxmsg2/5 -> Mux1/4
  raptor_can_rxmsg2/3 -> Mux1/2
  Demux1/1 -> raptor_data_write29/1
  Mux1/1 -> Demux1/1
  Demux1/4 -> raptor_data_write32/1
  raptor_can_rxmsg2/2 -> Mux1/1
  Demux1/3 -> raptor_data_write31/1
  Demux2/2 -> raptor_data_write23/1
  raptor_can_rxmsg8/4 -> Mux2/3
  raptor_can_rxmsg8/5 -> Mux2/4
  raptor_can_rxmsg8/3 -> Mux2/2
  Demux2/1 -> raptor_data_write22/1
  Mux2/1 -> Demux2/1
  Demux2/4 -> raptor_data_write25/1
  raptor_can_rxmsg8/2 -> Mux2/1
  Demux2/3 -> raptor_data_write24/1
  Demux3/2 -> raptor_data_write15/1
  raptor_can_rxmsg3/4 -> Mux3/3
  raptor_can_rxmsg3/5 -> Mux3/4
  raptor_can_rxmsg3/3 -> Mux3/2
  Demux3/1 -> raptor_data_write10/1
  Mux3/1 -> Demux3/1
  Demux3/4 -> raptor_data_write21/1
  raptor_can_rxmsg3/2 -> Mux3/1
  Demux3/3 -> raptor_data_write20/1
  Demux4/2 -> raptor_data_write2/1
  raptor_can_rxmsg4/4 -> Mux4/3
  raptor_can_rxmsg4/5 -> Mux4/4
  raptor_can_rxmsg4/3 -> Mux4/2
  Demux4/1 -> raptor_data_write1/1
  Mux4/1 -> Demux4/1
  Demux4/4 -> raptor_data_write4/1
  raptor_can_rxmsg4/2 -> Mux4/1
  Demux4/3 -> raptor_data_write3/1
  Demux5/2 -> raptor_data_write7/1
  raptor_can_rxmsg5/4 -> Mux5/3
  raptor_can_rxmsg5/5 -> Mux5/4
  raptor_can_rxmsg5/3 -> Mux5/2
  Demux5/1 -> raptor_data_write6/1
  Mux5/1 -> Demux5/1
  Demux5/4 -> raptor_data_write9/1
  raptor_can_rxmsg5/2 -> Mux5/1
  Demux5/3 -> raptor_data_write8/1
  Demux6/2 -> raptor_data_write12/1
  raptor_can_rxmsg6/4 -> Mux6/3
  raptor_can_rxmsg6/5 -> Mux6/4
  raptor_can_rxmsg6/3 -> Mux6/2
  Demux6/1 -> raptor_data_write11/1
  Mux6/1 -> Demux6/1
  Demux6/4 -> raptor_data_write14/1
  raptor_can_rxmsg6/2 -> Mux6/1
  Demux6/3 -> raptor_data_write13/1
  Demux7/2 -> raptor_data_write17/1
  raptor_can_rxmsg7/4 -> Mux7/3
  raptor_can_rxmsg7/5 -> Mux7/4
  raptor_can_rxmsg7/3 -> Mux7/2
  Demux7/1 -> raptor_data_write16/1
  Mux7/1 -> Demux7/1
  Demux7/4 -> raptor_data_write19/1
  raptor_can_rxmsg7/2 -> Mux7/1
  Demux7/3 -> raptor_data_write18/1
